simulink model "Model1"  (R2020a)
settings: Solver=VariableStepAuto  StartTime=0.0  StopTime=30  RelTol=1e-3
undefined symbols (not defined in the file or in its folder): a, a0, a1, a10, a11, a12, a13, a2, a3, a4, a5, a6, a7, a8, a9, b, camber, DiscIntNeverNeededParam, g, init_vel, init_y_pos, IT, max_vel, mT, mu_lateral, roadS1, roadS2, Ts
libraries: simulink x1
settings Model: PacingRate=0.800000  Creator=carmelo  LastModifiedBy=carmelo

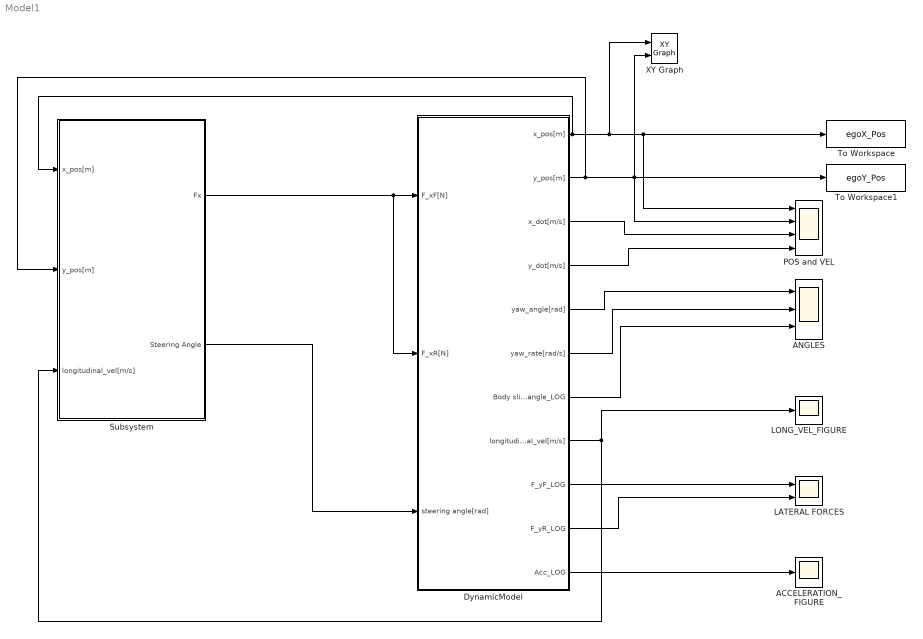
== system Model1 ==
  ACCELERATION_FIGURE : Scope
  ANGLES : Scope  NumInputPorts=3
  DynamicModel : Subsystem
  LATERAL FORCES : Scope  NumInputPorts=2
  LONG_VEL_FIGURE : Scope
  POS and VEL : Scope  NumInputPorts=4
  Subsystem : Subsystem
  To Workspace : ToWorkspace  VariableName=egoX_Pos  SampleTime=Ts
      settings: Decimation=3
  To Workspace1 : ToWorkspace  VariableName=egoY_Pos  SampleTime=Ts
      settings: Decimation=3
  XY Graph : simulink/Sinks/XY Graph  xmin=-800  xmax=800  ymin=-800  ymax=800  st=Ts
  wires:
  DynamicModel/3(x_dot[m/s]) -> POS and VEL/3
  DynamicModel/4(y_dot[m/s]) -> POS and VEL/4
  DynamicModel/5(yaw_angle[rad]) -> ANGLES/1
  DynamicModel/6(yaw_rate[rad/s]) -> ANGLES/2
  DynamicModel/8(longitudinal_vel[m/s]) -> LONG_VEL_FIGURE/1, Subsystem/3(longitudinal_vel[m/s])
  DynamicModel/9(F_yF_LOG) -> LATERAL FORCES/1
  DynamicModel/10(F_yR_LOG) -> LATERAL FORCES/2
  DynamicModel/7(Body slip angle_LOG) -> ANGLES/3
  DynamicModel/11(Acc_LOG) -> ACCELERATION_FIGURE/1
  DynamicModel/1(x_pos[m]) -> Subsystem/1(x_pos[m]), To Workspace/1, POS and VEL/1, XY Graph/1
  DynamicModel/2(y_pos[m]) -> Subsystem/2(y_pos[m]), POS and VEL/2, To Workspace1/1, XY Graph/2
  Subsystem/1(Fx) -> DynamicModel/1(F_xF[N]), DynamicModel/2(F_xR[N])
  Subsystem/2(Steering Angle) -> DynamicModel/3(steering angle[rad])

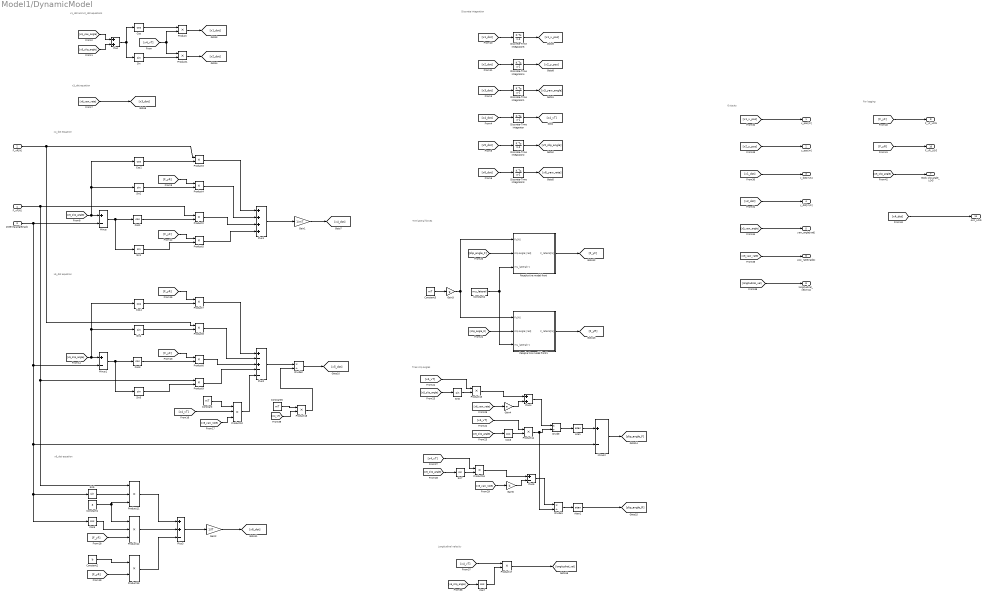
== system Model1/DynamicModel ==
  note: For logging
  note: Longitudinal velocity
  note: Outputs
  note: Tires slip angles
  note: Tire lateral forces
  note: x6_dot equation
  note: Discrete integration
  note: x4_dot equation
  note: x3_dot equation
  note: x1_dot and x2_dot equations
  note: x5_dot equation
  F_xF[N] : Inport  Unit=N
  F_xR[N] : Inport  Port=2  Unit=N
  steering angle[rad] : Inport  Port=3  Unit=rad
  Atan : Trigonometry  Operator=atan
  Atan1 : Trigonometry  Operator=atan
  Constant : Constant  Value=mT
  Constant1 : Constant  Value=a
  Constant2 : Constant  Value=b
  Constant3 : Constant  Value=mT
  Constant4 : Constant  Value=mu_lateral
  Constant5 : Constant  Value=mT
  Cos{,1..7} (8 alike) : Trigonometry  Operator=cos
  Discrete-Time Integrator : DiscreteIntegrator  InitialCondition=init_vel  SampleTime=Ts  ICPrevOutput=DiscIntNeverNeededParam  ICPrevScaledInput=DiscIntNeverNeededParam
  Discrete-Time Integrator{1..3,5} (4 alike) : DiscreteIntegrator  SampleTime=Ts  ICPrevOutput=DiscIntNeverNeededParam  ICPrevScaledInput=DiscIntNeverNeededParam
  Discrete-Time Integrator4 : DiscreteIntegrator  InitialCondition=init_y_pos;  SampleTime=Ts  ICPrevOutput=DiscIntNeverNeededParam  ICPrevScaledInput=DiscIntNeverNeededParam
  Divide : Product  Inputs=*/
  Divide1 : Product  Inputs=*/
  Divide2 : Product  Inputs=*/
  Gain1 : Gain  Gain=1/mT
  Gain2 : Gain  Gain=1/IT
  Gain3 : Gain  Gain=g
  Gain4 : Gain  Gain=a
  Gain5 : Gain  Gain=b
  Minus : Sum  Inputs=+-
  Minus1 : Sum  Inputs=+-
  Minus2 : Sum  Inputs=+-
  Pacejka tire model front : Subsystem
  Pacejka tire model front1 : Subsystem
  Plus : Sum
  Plus1 : Sum  Inputs=++++
  Plus2 : Sum  Inputs=+-+--
  Plus3 : Sum  Inputs=++-
  Plus4 : Sum
  Plus5 : Sum  Inputs=+-
  Product{,1..9,13..18} (16 alike) : Product
  Product10 : Product  Inputs=3
  Product11 : Product  Inputs=3
  Product12 : Product  Inputs=3
  Sin{,1..7} (8 alike) : Trigonometry
  x_pos[m] : Outport  Unit=m
  y_pos[m] : Outport  Port=2  Unit=m
  x_dot[m/s] : Outport  Port=3  Unit=m/s
  y_dot[m/s] : Outport  Port=4  Unit=m/s
  yaw_angle[rad] : Outport  Port=5  Unit=rad
  yaw_rate[rad/s] : Outport  Port=6  Unit=rad/s
  Body slip angle_LOG : Outport  Port=7  Unit=rad
  longitudinal_vel[m/s] : Outport  Port=8  Unit=m/s
  F_yF_LOG : Outport  Port=9  Unit=N
  F_yR_LOG : Outport  Port=10  Unit=N
  Acc_LOG : Outport  Port=11  Unit=m/s
  wires:
  Pacejka tire model front/1(F_lateral[N]) -> [F_yF]
  [x5_slip_angle] -> Sin7/1
  [x4_vT] -> Product16/1
  Atan/1 -> Minus2/1
  Product17/1 -> [longitudinal_vel]
  [x1_x_pos] -> x_pos[m]/1
  [x6_yaw_rate] -> Gain4/1
  [F_yR] -> Product13/2
  Pacejka tire model front1/1(F_lateral[N]) -> [F_yR]
  Sin/1 -> Product1/2
  Discrete-Time Integrator/1 -> [x4_vT]
  Cos7/1 -> Product17/2
  Sin2/1 -> Product4/2
  Product4/1 -> Plus1/2
  [x3_dot] -> Discrete-Time Integrator1/1
  Divide1/1 -> Atan1/1
  Product2/1 -> Plus1/3
  [F_yF] -> Product6/1
  Product14/1 -> Divide/2, Divide1/2
  [x5_slip_angle] -> Sin2/1, Cos2/1, Minus/1
  Minus2/1 -> [slip_angle_F]
  Cos2/1 -> Product3/2
  [x5_slip_angle] -> Plus/2
  Sin7/1 -> Product16/2
  Constant4/1 -> Pacejka tire model front/3(mu_lateral[-]), Pacejka tire model front1/3(mu_lateral[-])
  Discrete-Time Integrator3/1 -> [x6_yaw_rate]
  [x4_dot] -> Discrete-Time Integrator/1
  Product/1 -> [x1_dot]
  [x3_yaw_angle] -> yaw_angle[rad]/1
  [x1_dot] -> x_dot[m/s]/1
  F_xR[N]/1 -> Product3/1, Product8/1
  Constant2/1 -> Product13/1
  Cos3/1 -> Product6/2
  [x2_dot] -> Discrete-Time Integrator4/1
  Minus/1 -> Sin1/1, Cos1/1
  [slip_angle_R] -> Pacejka tire model front1/2(slip angle [rad])
  Gain3/1 -> Pacejka tire model front1/1(Fz[N]), Pacejka tire model front/1(Fz[N])
  [x6_dot] -> Discrete-Time Integrator3/1
  Discrete-Time Integrator1/1 -> [x3_yaw_angle]
  Gain4/1 -> Plus4/2
  Constant3/1 -> Gain3/1
  [x2_y_pos] -> y_pos[m]/1
  Cos1/1 -> Product2/2
  Gain2/1 -> [x6_dot]
  [x4_vT] -> Product10/2
  [x6_yaw_rate] -> [x3_dot]
  [F_yF] -> Product5/1
  [x3_yaw_angle] -> Plus/1
  [x6_yaw_rate] -> yaw_rate[rad/s]/1
  [F_yR] -> Product4/1
  [slip_angle_F] -> Pacejka tire model front/2(slip angle [rad])
  [x4_vT] -> Product15/1
  [longitudinal_vel] -> longitudinal_vel[m/s]/1
  [x5_slip_angle] -> Sin6/1
  Product11/1 -> Plus3/1
  [F_yR] -> Product7/1
  Atan1/1 -> [slip_angle_R]
  Divide/1 -> Atan/1
  [x4_vT] -> Product1/1, Product/2
  Product1/1 -> [x2_dot]
  Cos4/1 -> Product7/2
  Sin5/1 -> Product11/2
  Plus5/1 -> Divide1/1
  [x5_slip_angle] -> Cos6/1
  Sin4/1 -> Product8/2
  [x6_yaw_rate] -> Product10/3
  Cos5/1 -> Product12/2
  Plus3/1 -> Gain2/1
  Cos/1 -> Product/1
  Product13/1 -> Plus3/3
  Cos6/1 -> Product14/2
  F_xF[N]/1 -> Product9/1, Product11/1, Product2/1
  Discrete-Time Integrator5/1 -> [x1_x_pos]
  Plus/1 -> Cos/1, Sin/1
  Product12/1 -> Plus3/2
  Product5/1 -> Plus1/4
  steering angle[rad]/1 -> Minus2/2, Cos5/1, Sin5/1, Minus1/2, Minus/2
  Product15/1 -> Plus4/1
  [x5_dot] -> Discrete-Time Integrator2/1
  Product9/1 -> Plus2/4
  Product16/1 -> Plus5/1
  [x4_vT] -> Product14/1
  Constant/1 -> Product10/1
  [x4_vT] -> Product17/1
  Sin3/1 -> Product9/2
  Plus2/1 -> Divide2/1
  Product6/1 -> Plus2/3
  [x5_slip_angle] -> Sin4/1, Cos4/1, Minus1/1
  Constant1/1 -> Product11/3, Product12/1
  Divide2/1 -> [x5_dot]
  Discrete-Time Integrator4/1 -> [x2_y_pos]
  [F_yF] -> Product12/3
  Minus1/1 -> Sin3/1, Cos3/1
  Product10/1 -> Plus2/5
  Product7/1 -> Plus2/1
  [x5_slip_angle] -> Cos7/1
  Sin1/1 -> Product5/2
  [x6_yaw_rate] -> Gain5/1
  [x1_dot] -> Discrete-Time Integrator5/1
  [x2_dot] -> y_dot[m/s]/1
  Product3/1 -> Plus1/1
  Sin6/1 -> Product15/2
  Discrete-Time Integrator2/1 -> [x5_slip_angle]
  Product8/1 -> Plus2/2
  Plus4/1 -> Divide/1
  Gain5/1 -> Plus5/2
  Gain1/1 -> [x4_dot]
  Plus1/1 -> Gain1/1
  [F_yF] -> F_yF_LOG/1
  [F_yR] -> F_yR_LOG/1
  [x5_slip_angle] -> Body slip angle_LOG/1
  [x4_dot] -> Acc_LOG/1
  Product18/1 -> Divide2/2
  Constant5/1 -> Product18/1
  [x4_vT] -> Product18/2

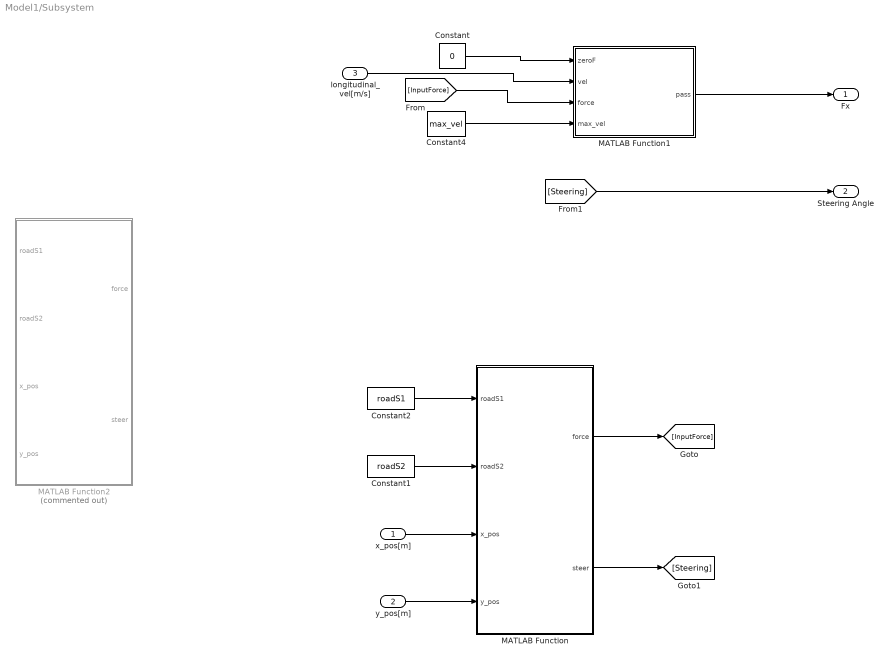
== system Model1/Subsystem ==
  x_pos[m] : Inport
  y_pos[m] : Inport  Port=2
  longitudinal_vel[m/s] : Inport  Port=3
  Constant : Constant  Value=0
  Constant1 : Constant  Value=roadS2  VectorParams1D=off
  Constant2 : Constant  Value=roadS1  VectorParams1D=off
  Constant4 : Constant  Value=max_vel
  MATLAB Function : MATLAB Function  TreatAsAtomicUnit=on
  MATLAB Function1 : MATLAB Function  TreatAsAtomicUnit=on
  MATLAB Function2 : MATLAB Function  Commented=on  TreatAsAtomicUnit=on
  Fx : Outport  Unit=N
  Steering Angle : Outport  Port=2  Unit=rad
  wires:
  [Steering] -> Steering Angle/1
  longitudinal_vel[m/s]/1 -> MATLAB Function1/2(vel)
  Constant/1 -> MATLAB Function1/1(zeroF)
  MATLAB Function1/1(pass) -> Fx/1
  [InputForce] -> MATLAB Function1/3(force)
  MATLAB Function/1(force) -> [InputForce]
  x_pos[m]/1 -> MATLAB Function/3(x_pos)
  y_pos[m]/1 -> MATLAB Function/4(y_pos)
  Constant2/1 -> MATLAB Function/1(roadS1)
  MATLAB Function/2(steer) -> [Steering]
  Constant1/1 -> MATLAB Function/2(roadS2)
  Constant4/1 -> MATLAB Function1/4(max_vel)

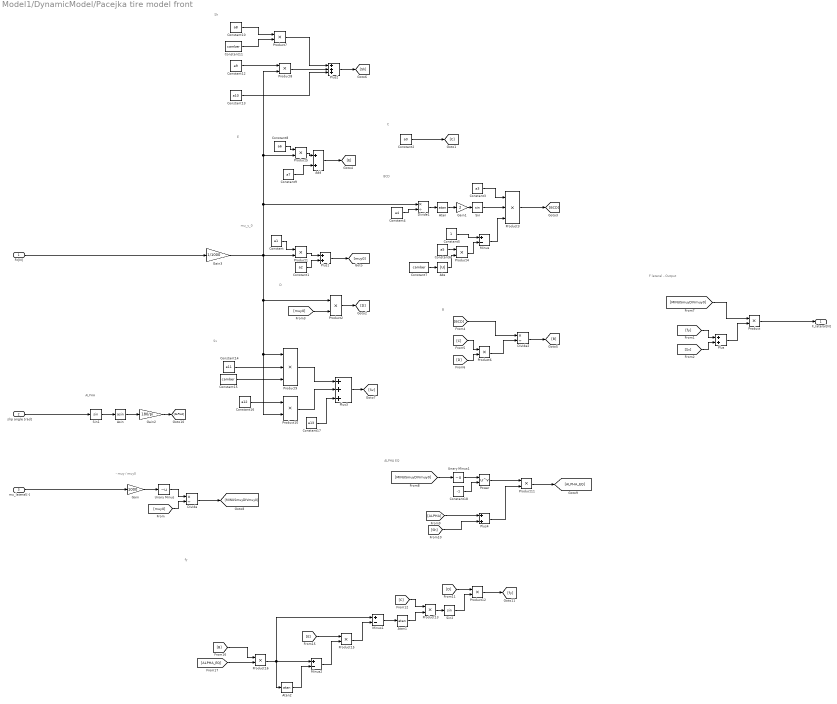
== system Model1/DynamicModel/Pacejka tire model front ==
  note: fy
  note: ALPHA
  note: - muy / muy0
  note: ALPHA EQ
  note: Sv
  note: Sh
  note: B
  note: E
  note: BCD
  note: C
  note: D
  note: mu_y_0
  note: F lateral - Output
  Fz[N] : Inport  Unit=N
  slip angle [rad] : Inport  Port=2  Unit=rad
  mu_lateral[-] : Inport  Port=3
  Abs : Abs
  Add : Sum
  Asin : Trigonometry  Operator=asin
  Atan : Trigonometry  Operator=atan
  Atan1 : Trigonometry  Operator=atan
  Atan2 : Trigonometry  Operator=atan
  Constant : Constant  Value=a1
  Constant1 : Constant  Value=a2
  Constant10 : Constant  Value=a8
  Constant11 : Constant  Value=camber
  Constant12 : Constant  Value=a9
  Constant13 : Constant  Value=a10
  Constant14 : Constant  Value=a11
  Constant15 : Constant  Value=camber
  Constant16 : Constant  Value=a12
  Constant17 : Constant  Value=a13
  Constant18 : Constant  Value=-1
  Constant2 : Constant  Value=a0
  Constant3 : Constant  Value=a3
  Constant4 : Constant  Value=a4
  Constant5 : Constant
  Constant6 : Constant  Value=a5
  Constant7 : Constant  Value=camber
  Constant8 : Constant  Value=a6
  Constant9 : Constant  Value=a7
  Divide : Product  Inputs=*/
  Divide1 : Product  Inputs=*/
  Divide2 : Product  Inputs=*/
  Gain : Gain  Gain=1000
  Gain1 : Gain  Gain=2
  Gain2 : Gain  Gain=180/pi
  Gain3 : Gain  Gain=1/1000
  Minus : Sum  Inputs=+-
  Minus1 : Sum  Inputs=+-
  Minus2 : Sum  Inputs=+-
  Plus : Sum
  Plus1 : Sum
  Plus2 : Sum  Inputs=+++
  Plus3 : Sum  Inputs=+++
  Plus4 : Sum
  Power : Math  Operator=pow  SaturateOnIntegerOverflow=on
  Product{,1..2,4..8,10..13,15..16} (14 alike) : Product
  Product3 : Product  Inputs=3
  Product9 : Product  Inputs=3
  Sin : Trigonometry
  Sin1 : Trigonometry
  Sin2 : Trigonometry
  Unary Minus : UnaryMinus
  Unary Minus1 : UnaryMinus
  F_lateral[N] : Outport  Unit=N
  wires:
  Unary Minus/1 -> Divide/1
  Product7/1 -> Plus2/1
  Sin/1 -> Product3/2
  Constant9/1 -> Add/2
  Asin/1 -> Gain2/1
  Constant8/1 -> Product5/1
  Constant4/1 -> Divide1/2
  Constant10/1 -> Product7/1
  Constant13/1 -> Plus2/3
  Product4/1 -> Minus/2
  [fy] -> Plus/1
  Add/1 -> [E]
  Atan2/1 -> Minus2/2
  Constant3/1 -> Product3/1
  Gain1/1 -> Sin/1
  Sin2/1 -> Product12/2
  Constant15/1 -> Product9/3
  Abs/1 -> Product4/2
  [BCD] -> Divide2/1
  Constant5/1 -> Minus/1
  [D] -> Product12/1
  Product2/1 -> [D]
  Constant6/1 -> Product4/1
  [Sv] -> Plus/2
  Divide1/1 -> Atan/1
  Product8/1 -> Plus2/2
  Fz[N]/1 -> Gain3/1
  Product16/1 -> Minus1/1, Atan2/1, Minus2/1
  Sin1/1 -> Asin/1
  Plus4/1 -> Product11/2
  [C] -> Product6/1
  Product3/1 -> [BCD]
  Product9/1 -> Plus3/1
  Constant17/1 -> Plus3/3
  Product6/1 -> Divide2/2
  Product13/1 -> Sin2/1
  Gain2/1 -> [ALPHA]
  Product12/1 -> [fy]
  Plus2/1 -> [Sh]
  Plus1/1 -> [muy0]
  mu_lateral[-]/1 -> Gain/1
  [ALPHA_EQ] -> Product16/2
  Product10/1 -> Plus3/2
  [MINUSmuyDIVmuy0] -> Product/1
  [muy0] -> Product2/2
  [ALPHA] -> Plus4/1
  [D] -> Product6/2
  Constant/1 -> Product1/1
  Gain3/1 -> Divide1/1, Product5/2, Product8/2, Product1/2, Product2/1, Product9/1, Product10/2
  Unary Minus1/1 -> Power/1
  Constant18/1 -> Power/2
  Product5/1 -> Add/1
  Minus1/1 -> Atan1/1
  [E] -> Product15/1
  [Sh] -> Plus4/2
  Plus/1 -> Product/2
  Constant11/1 -> Product7/2
  Plus3/1 -> [Sv]
  Product/1 -> F_lateral[N]/1
  Constant1/1 -> Plus1/2
  Power/1 -> Product11/1
  Atan1/1 -> Product13/2
  [muy0] -> Divide/2
  Product15/1 -> Minus1/2
  Constant14/1 -> Product9/2
  Constant2/1 -> [C]
  Divide/1 -> [MINUSmuyDIVmuy0]
  Gain/1 -> Unary Minus/1
  Product11/1 -> [ALPHA_EQ]
  Constant16/1 -> Product10/1
  Atan/1 -> Gain1/1
  Constant7/1 -> Abs/1
  [MINUSmuyDIVmuy0] -> Unary Minus1/1
  Constant12/1 -> Product8/1
  [C] -> Product13/1
  Minus2/1 -> Product15/2
  slip angle [rad]/1 -> Sin1/1
  Divide2/1 -> [B]
  Product1/1 -> Plus1/1
  Minus/1 -> Product3/3
  [B] -> Product16/1

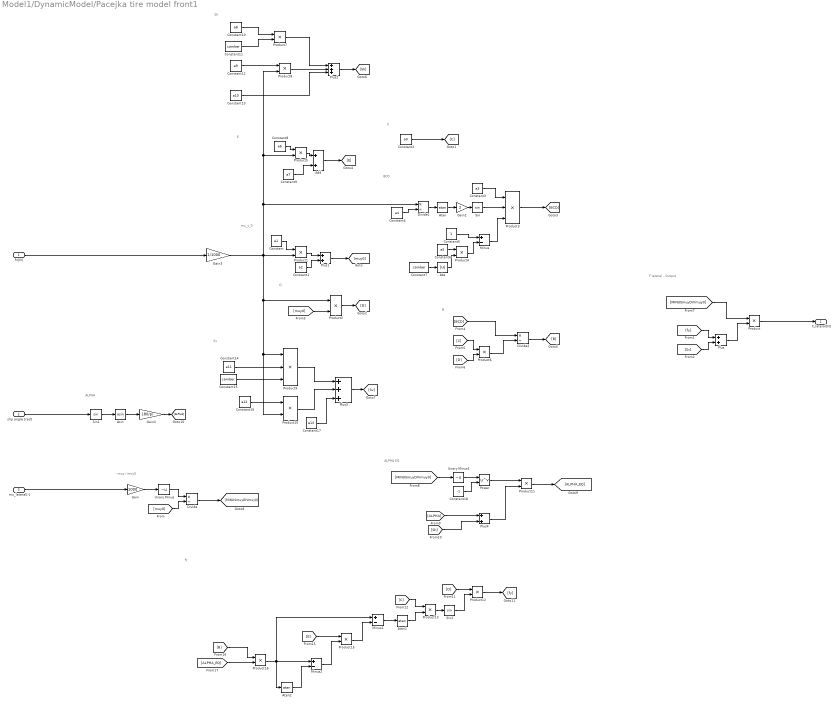
== system Model1/DynamicModel/Pacejka tire model front1 ==
  note: fy
  note: ALPHA
  note: - muy / muy0
  note: ALPHA EQ
  note: Sv
  note: Sh
  note: B
  note: E
  note: BCD
  note: C
  note: D
  note: mu_y_0
  note: F lateral - Output
  Fz[N] : Inport  Unit=N
  slip angle [rad] : Inport  Port=2  Unit=rad
  mu_lateral[-] : Inport  Port=3
  Abs : Abs
  Add : Sum
  Asin : Trigonometry  Operator=asin
  Atan : Trigonometry  Operator=atan
  Atan1 : Trigonometry  Operator=atan
  Atan2 : Trigonometry  Operator=atan
  Constant : Constant  Value=a1
  Constant1 : Constant  Value=a2
  Constant10 : Constant  Value=a8
  Constant11 : Constant  Value=camber
  Constant12 : Constant  Value=a9
  Constant13 : Constant  Value=a10
  Constant14 : Constant  Value=a11
  Constant15 : Constant  Value=camber
  Constant16 : Constant  Value=a12
  Constant17 : Constant  Value=a13
  Constant18 : Constant  Value=-1
  Constant2 : Constant  Value=a0
  Constant3 : Constant  Value=a3
  Constant4 : Constant  Value=a4
  Constant5 : Constant
  Constant6 : Constant  Value=a5
  Constant7 : Constant  Value=camber
  Constant8 : Constant  Value=a6
  Constant9 : Constant  Value=a7
  Divide : Product  Inputs=*/
  Divide1 : Product  Inputs=*/
  Divide2 : Product  Inputs=*/
  Gain : Gain  Gain=1000
  Gain1 : Gain  Gain=2
  Gain2 : Gain  Gain=180/pi
  Gain3 : Gain  Gain=1/1000
  Minus : Sum  Inputs=+-
  Minus1 : Sum  Inputs=+-
  Minus2 : Sum  Inputs=+-
  Plus : Sum
  Plus1 : Sum
  Plus2 : Sum  Inputs=+++
  Plus3 : Sum  Inputs=+++
  Plus4 : Sum
  Power : Math  Operator=pow  SaturateOnIntegerOverflow=on
  Product{,1..2,4..8,10..13,15..16} (14 alike) : Product
  Product3 : Product  Inputs=3
  Product9 : Product  Inputs=3
  Sin : Trigonometry
  Sin1 : Trigonometry
  Sin2 : Trigonometry
  Unary Minus : UnaryMinus
  Unary Minus1 : UnaryMinus
  F_lateral[N] : Outport  Unit=N
  wires:
  Unary Minus/1 -> Divide/1
  Product7/1 -> Plus2/1
  Sin/1 -> Product3/2
  Constant9/1 -> Add/2
  Asin/1 -> Gain2/1
  Constant8/1 -> Product5/1
  Constant4/1 -> Divide1/2
  Constant10/1 -> Product7/1
  Constant13/1 -> Plus2/3
  Product4/1 -> Minus/2
  [fy] -> Plus/1
  Add/1 -> [E]
  Atan2/1 -> Minus2/2
  Constant3/1 -> Product3/1
  Gain1/1 -> Sin/1
  Sin2/1 -> Product12/2
  Constant15/1 -> Product9/3
  Abs/1 -> Product4/2
  [BCD] -> Divide2/1
  Constant5/1 -> Minus/1
  [D] -> Product12/1
  Product2/1 -> [D]
  Constant6/1 -> Product4/1
  [Sv] -> Plus/2
  Divide1/1 -> Atan/1
  Product8/1 -> Plus2/2
  Fz[N]/1 -> Gain3/1
  Product16/1 -> Minus1/1, Atan2/1, Minus2/1
  Sin1/1 -> Asin/1
  Plus4/1 -> Product11/2
  [C] -> Product6/1
  Product3/1 -> [BCD]
  Product9/1 -> Plus3/1
  Constant17/1 -> Plus3/3
  Product6/1 -> Divide2/2
  Product13/1 -> Sin2/1
  Gain2/1 -> [ALPHA]
  Product12/1 -> [fy]
  Plus2/1 -> [Sh]
  Plus1/1 -> [muy0]
  mu_lateral[-]/1 -> Gain/1
  [ALPHA_EQ] -> Product16/2
  Product10/1 -> Plus3/2
  [MINUSmuyDIVmuy0] -> Product/1
  [muy0] -> Product2/2
  [ALPHA] -> Plus4/1
  [D] -> Product6/2
  Constant/1 -> Product1/1
  Gain3/1 -> Divide1/1, Product5/2, Product8/2, Product1/2, Product2/1, Product9/1, Product10/2
  Unary Minus1/1 -> Power/1
  Constant18/1 -> Power/2
  Product5/1 -> Add/1
  Minus1/1 -> Atan1/1
  [E] -> Product15/1
  [Sh] -> Plus4/2
  Plus/1 -> Product/2
  Constant11/1 -> Product7/2
  Plus3/1 -> [Sv]
  Product/1 -> F_lateral[N]/1
  Constant1/1 -> Plus1/2
  Power/1 -> Product11/1
  Atan1/1 -> Product13/2
  [muy0] -> Divide/2
  Product15/1 -> Minus1/2
  Constant14/1 -> Product9/2
  Constant2/1 -> [C]
  Divide/1 -> [MINUSmuyDIVmuy0]
  Gain/1 -> Unary Minus/1
  Product11/1 -> [ALPHA_EQ]
  Constant16/1 -> Product10/1
  Atan/1 -> Gain1/1
  Constant7/1 -> Abs/1
  [MINUSmuyDIVmuy0] -> Unary Minus1/1
  Constant12/1 -> Product8/1
  [C] -> Product13/1
  Minus2/1 -> Product15/2
  slip angle [rad]/1 -> Sin1/1
  Divide2/1 -> [B]
  Product1/1 -> Plus1/1
  Minus/1 -> Product3/3
  [B] -> Product16/1

== matlab function Model1/Subsystem/MATLAB Function1 ==
  data: zeroF input; vel input; pass output; force input; max_vel input
function pass = mySwitch(zeroF, vel, force, max_vel)

if vel > max_vel && force > 0
    pass = zeroF; 
elseif vel < 0 && force < 0
    pass = zeroF;
else
    pass = force;
end

== matlab function Model1/Subsystem/MATLAB Function ==
  data: roadS1 input; roadS2 input; x_pos input; force output; y_pos input; steer output
function [force, steer] = ...
    calculateForce(roadS1, roadS2, x_pos, y_pos)

max_force = 2200;
min_force = -2000;
curve_force = 0;
curve_steer = 0.085;

brake_offset1 = 160;
brake_offset2 = 20; 

steer_offset = 40;

% does not consider that force cannot be applied "as an impulse"

if x_pos > roadS1(1,1) + brake_offset1 && x_pos <  roadS1(1,2) - brake_offset1
    % first or third long straight sectors
    force = max_force;
    steer = 0;
    
elseif (x_pos < roadS1(1,1) + brake_offset1 && x_pos > roadS1(1,1)) || ...
        (x_pos > roadS1(1,2) - brake_offset1 && x_pos < roadS1(1,2))
    % brake in long straight
    force = min_force;
    steer = 0.004;
    
elseif y_pos > roadS2(2,1) + brake_offset2 && y_pos < roadS2(2,2) - brake_offset2
    % second and fourth short straight sectors
    force = max_force;
    steer = 0;

elseif (y_pos < roadS2(2,1) + brake_offset2 && y_pos > roadS2(2,1)) || ...
        (y_pos > roadS2(2,2) - brake_offset2 && y_pos < roadS2(2,2))
    % brake in short straight
    force = min_force;
    steer = -0.015;
    
else
    if x_pos >= roadS1(1,2) && x_pos < roadS1(1,2) + steer_offset && y_pos < roadS2(2,1)
        %beginning of first curve
        force = min_force/4;
        steer = 0.06;
    
    elseif y_pos < roadS2(2,1) && y_pos > roadS2(2,1) - steer_offset && x_pos > roadS1(1,2)
        %%end of first curve
        force = max_force/5;
        steer = 0;
        
    else
        %curves
        force = curve_force;
        steer = curve_steer;
    
    end
end

== matlab function Model1/Subsystem/MATLAB Function2 ==
  data: roadS1 input; roadS2 input; x_pos input; force output; y_pos input; steer output
function [force, steer] = ...
    calculateForce(roadS1, roadS2, x_pos, y_pos)

max_force = 2200;
min_force = -2000;
curve_force = 0;
curve_steer = 0.08;

brake_offset1 = 160;
brake_offset2 = 20; 

% does not consider that force cannot be applied "as an impulse"

if x_pos > roadS1(1,1) + brake_offset1 && x_pos <  roadS1(1,2) - brake_offset1
    % first or third long straight sectors
    force = max_force;
    steer = 0;
    
elseif (x_pos < roadS1(1,1) + brake_offset1 && x_pos > roadS1(1,1)) || ...
        (x_pos > roadS1(1,2) - brake_offset1 && x_pos < roadS1(1,2))
    % brake in long straight
    force = min_force;
    steer = 0.005;
    
elseif y_pos > roadS2(2,1) + brake_offset2 && y_pos < roadS2(2,2) - brake_offset2
    % second and fourth short straight sectors
    force = max_force;
    steer = 0;

elseif (y_pos < roadS2(2,1) + brake_offset2 && y_pos > roadS2(2,1)) || ...
        (y_pos > roadS2(2,2) - brake_offset2 && y_pos < roadS2(2,2))
    % brake in short straight
    force = min_force;
    steer = -0.01;
    
else
    % curves
    force = curve_force;
    steer = curve_steer;
    
end
